simulink model "validate_magnetometer"  (R2014a)
settings: Solver=VariableStepDiscrete  StartTime=0.0  StopTime=t_sim  MaxStep=0.001  RelTol=1e-3
undefined symbols (not defined in the file): acc_data, diff, gravity_I, magnetometer_data, R_acc, R_magnetometer, ref_B_I
libraries: lib_gyro_fusion x7
settings Model: Creator=kirill  LastModifiedBy=kirill

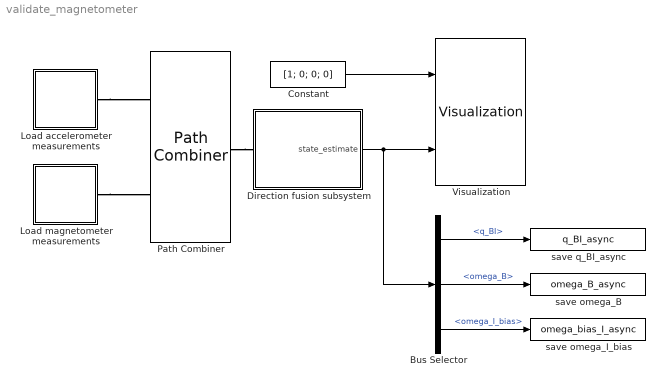
== system validate_magnetometer ==
  Bus Selector : BusSelector  OutputSignals=q_BI,omega_B,omega_I_bias
  Constant : Constant  Value=[1; 0; 0; 0]
  Direction fusion subsystem : Subsystem
  Load accelerometer measurements : Subsystem  mask{measurement_type=2, observed_data=acc_data, R_measurement=R_acc, ref_direction_I=gravity_I}
      mask prompts: measurement_type "Measuerment type (integer identifyer)"; observed_data "Observation data (see from workspace documentation)"; R_measurement "Measurement covariance matrix"; ref_direction_I "Reference direction"
  Load magnetometer measurements : Subsystem  mask{measurement_type=2, observed_data=magnetometer_data, R_measurement=R_magnetometer, ref_direction_I=ref_B_I}
      mask prompts: measurement_type "Measuerment type (integer identifyer)"; observed_data "Observation data (see from workspace documentation)"; R_measurement "Measurement covariance matrix"; ref_direction_I "Reference direction"
  Path Combiner : PathCombiner  NumberInputPorts=2
  Visualization : lib_gyro_fusion/Visualization
  save omega_B : ToWorkspace  VariableName=omega_B_async  SaveFormat=Timeseries  SampleTime=-1
  save omega_I_bias : ToWorkspace  VariableName=omega_bias_I_async  SaveFormat=Timeseries  SampleTime=-1
  save q_BI_async : ToWorkspace  VariableName=q_BI_async  SaveFormat=Timeseries  SampleTime=-1
  wires:
  Direction fusion subsystem/1(state_estimate) -> Visualization/2, Bus Selector/1
  Constant/1 -> Visualization/1
  Bus Selector/1 -> save q_BI_async/1  "<q_BI>"
  Bus Selector/3 -> save omega_I_bias/1  "<omega_I_bias>"
  Bus Selector/2 -> save omega_B/1  "<omega_B>"
  connections:
  Load accelerometer measurements/RConn1 -- Path Combiner/LConn1
  Path Combiner/RConn1 -- Direction fusion subsystem/LConn1
  Load magnetometer measurements/RConn1 -- Path Combiner/LConn2

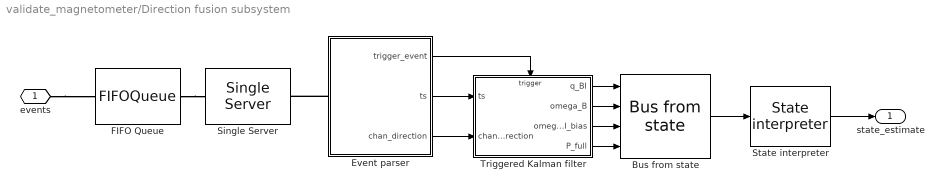
== system validate_magnetometer/Direction fusion subsystem ==
  Bus from state : lib_gyro_fusion/Bus from state
  Event parser : Subsystem
  FIFO Queue : FIFOQueue  Capacity=500
  Single Server : SingleServer  ServiceTime=0.001
  State interpreter : lib_gyro_fusion/State interpreter
  Triggered Kalman filter : Subsystem  TreatAsAtomicUnit=on
  events : PMIOPort  Port=1  Side=Left
  state_estimate : Outport
  wires:
  Event parser/3(chan_direction) -> Triggered Kalman filter/2(chan_direction)
  Event parser/1(trigger_event) -> Triggered Kalman filter/Trigger
  Event parser/2(ts) -> Triggered Kalman filter/1(ts)
  Bus from state/1 -> State interpreter/1
  State interpreter/1 -> state_estimate/1
  Triggered Kalman filter/1(q_BI) -> Bus from state/1
  Triggered Kalman filter/2(omega_B) -> Bus from state/2
  Triggered Kalman filter/3(omega_I_bias) -> Bus from state/3
  Triggered Kalman filter/4(P_full) -> Bus from state/4
  connections:
  events/RConn1 -- FIFO Queue/LConn1
  FIFO Queue/RConn1 -- Single Server/LConn1
  Event parser/LConn1 -- Single Server/RConn1

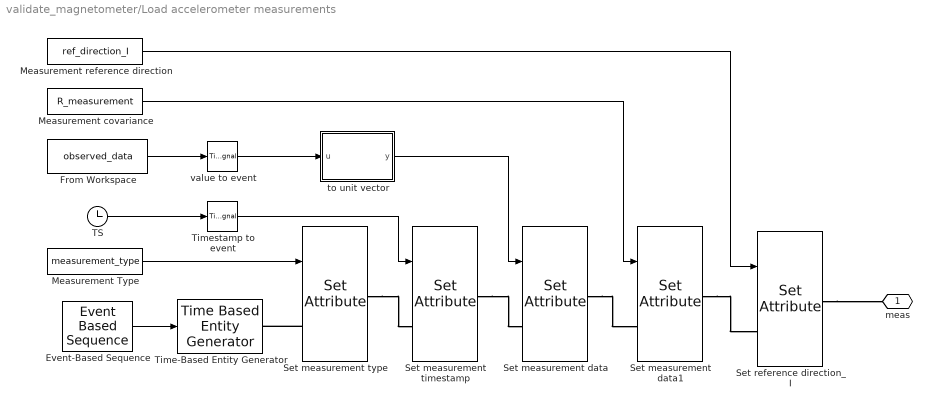
== system validate_magnetometer/Load accelerometer measurements ==
  Event-Based Sequence : EventBasedSequence  VectorOutputValues=diff(observed_data.time)  FormOutputOpt=Setting to infinity
  From Workspace : FromWorkspace  VariableName=observed_data  SampleTime=0
  Measurement Type : Constant  Value=measurement_type
  Measurement covariance : Constant  Value=R_measurement
  Measurement reference direction : Constant  Value=ref_direction_I
  Set measurement data : SetAttribute  AttributeName=value  AttributeFrom=Signal port  EvaluatedAttributeValue={ []}
  Set measurement data1 : SetAttribute  AttributeName=R  AttributeFrom=Signal port  EvaluatedAttributeValue={ []}
  Set measurement timestamp : SetAttribute  AttributeName=ts  AttributeFrom=Signal port  EvaluatedAttributeValue={ []}
  Set measurement type : SetAttribute  AttributeName=meas_type  AttributeFrom=Signal port  EvaluatedAttributeValue={ []}
  Set reference direction_I : SetAttribute  AttributeName=ref_direction_I  AttributeFrom=Signal port  EvaluatedAttributeValue={ []}
  TS : Clock
  Time-Based Entity Generator : TimeBasedEntityGenerator  GenerateEntitiesUpon=Intergeneration time from port t
  Timestamp to event : TimedToEventSignal
  to unit vector : MATLAB Function  TreatAsAtomicUnit=on
  value to event : TimedToEventSignal
  meas : PMIOPort  Port=1  Side=Right
  wires:
  TS/1 -> Timestamp to event/1
  From Workspace/1 -> value to event/1
  Event-Based Sequence/1 -> Time-Based Entity Generator/1
  Measurement Type/1 -> Set measurement type/1
  Timestamp to event/1 -> Set measurement timestamp/1
  value to event/1 -> to unit vector/1(u)
  Measurement covariance/1 -> Set measurement data1/1
  Measurement reference direction/1 -> Set reference direction_I/1
  to unit vector/1(y) -> Set measurement data/1
  connections:
  Set measurement type/LConn1 -- Time-Based Entity Generator/RConn1
  Set measurement type/RConn1 -- Set measurement timestamp/LConn1
  Set measurement timestamp/RConn1 -- Set measurement data/LConn1
  Set measurement data/RConn1 -- Set measurement data1/LConn1
  Set measurement data1/RConn1 -- Set reference direction_I/LConn1
  Set reference direction_I/RConn1 -- meas/RConn1

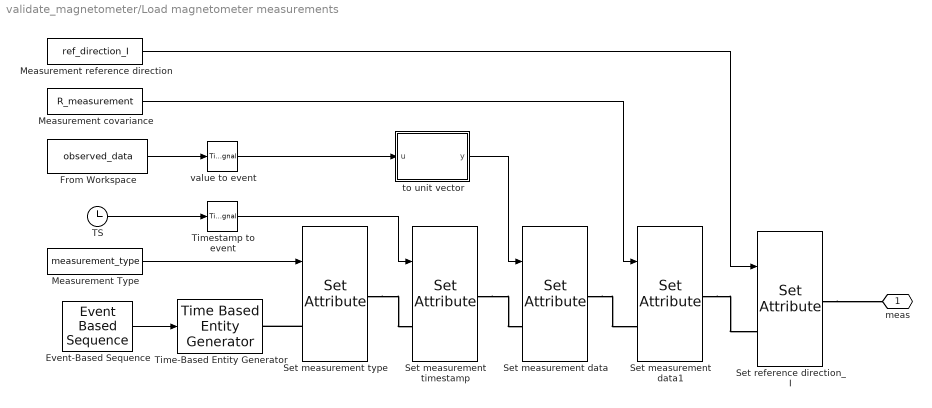
== system validate_magnetometer/Load magnetometer measurements ==
  Event-Based Sequence : EventBasedSequence  VectorOutputValues=diff(observed_data.time)  FormOutputOpt=Setting to infinity
  From Workspace : FromWorkspace  VariableName=observed_data  SampleTime=0
  Measurement Type : Constant  Value=measurement_type
  Measurement covariance : Constant  Value=R_measurement
  Measurement reference direction : Constant  Value=ref_direction_I
  Set measurement data : SetAttribute  AttributeName=value  AttributeFrom=Signal port  EvaluatedAttributeValue={ []}
  Set measurement data1 : SetAttribute  AttributeName=R  AttributeFrom=Signal port  EvaluatedAttributeValue={ []}
  Set measurement timestamp : SetAttribute  AttributeName=ts  AttributeFrom=Signal port  EvaluatedAttributeValue={ []}
  Set measurement type : SetAttribute  AttributeName=meas_type  AttributeFrom=Signal port  EvaluatedAttributeValue={ []}
  Set reference direction_I : SetAttribute  AttributeName=ref_direction_I  AttributeFrom=Signal port  EvaluatedAttributeValue={ []}
  TS : Clock
  Time-Based Entity Generator : TimeBasedEntityGenerator  GenerateEntitiesUpon=Intergeneration time from port t
  Timestamp to event : TimedToEventSignal
  to unit vector : MATLAB Function  TreatAsAtomicUnit=on
  value to event : TimedToEventSignal
  meas : PMIOPort  Port=1  Side=Right
  wires:
  TS/1 -> Timestamp to event/1
  From Workspace/1 -> value to event/1
  Event-Based Sequence/1 -> Time-Based Entity Generator/1
  Measurement Type/1 -> Set measurement type/1
  Timestamp to event/1 -> Set measurement timestamp/1
  value to event/1 -> to unit vector/1(u)
  Measurement covariance/1 -> Set measurement data1/1
  Measurement reference direction/1 -> Set reference direction_I/1
  to unit vector/1(y) -> Set measurement data/1
  connections:
  Set measurement type/LConn1 -- Time-Based Entity Generator/RConn1
  Set measurement type/RConn1 -- Set measurement timestamp/LConn1
  Set measurement timestamp/RConn1 -- Set measurement data/LConn1
  Set measurement data/RConn1 -- Set measurement data1/LConn1
  Set measurement data1/RConn1 -- Set reference direction_I/LConn1
  Set reference direction_I/RConn1 -- meas/RConn1

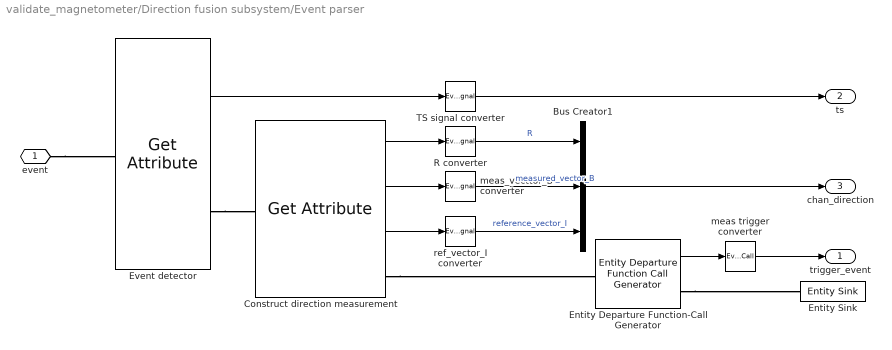
== system validate_magnetometer/Direction fusion subsystem/Event parser ==
  Bus Creator1 : BusCreator  Inputs=3
  Construct direction measurement : GetAttribute  AttributeName=R|value|ref_direction_I  AttributeMissing=Error|Error|Error  AttributeDefaultValue=1|1|1  AttributeTreatAsVector=1|1|1  AttributeSendTiming=After entity departure|After entity departure|After entity departure  EvaluatedDefaultAttributeValue={ [];[];[]}
      settings: OutputPortMap=o1,o2,o3
  Entity Departure Function-Call Generator : EntityDepartureFunctionCallGenerator
  Entity Sink : EntitySink
  Event detector : GetAttribute  AttributeName=ts  EvaluatedDefaultAttributeValue={ []}
      settings: OutputPortMap=o1
  R converter : EventToTimedSignal
  TS signal converter : EventToTimedSignal
  meas trigger converter : EventToTimedFunctionCall
  meas_vecttor_B converter : EventToTimedSignal
  ref_vector_I converter : EventToTimedSignal
  event : PMIOPort  Port=1  Side=Left
  trigger_event : Outport
  ts : Outport  Port=2
  chan_direction : Outport  Port=3
  wires:
  Construct direction measurement/1 -> R converter/1
  Bus Creator1/1 -> chan_direction/1
  Construct direction measurement/2 -> meas_vecttor_B converter/1
  ref_vector_I converter/1 -> Bus Creator1/3  "reference_vector_I"
  R converter/1 -> Bus Creator1/1  "R"
  meas_vecttor_B converter/1 -> Bus Creator1/2  "measured_vector_B"
  Construct direction measurement/3 -> ref_vector_I converter/1
  Entity Departure Function-Call Generator/1 -> meas trigger converter/1
  meas trigger converter/1 -> trigger_event/1
  TS signal converter/1 -> ts/1
  Event detector/1 -> TS signal converter/1
  connections:
  Entity Departure Function-Call Generator/RConn1 -- Entity Sink/LConn1
  Construct direction measurement/RConn1 -- Entity Departure Function-Call Generator/LConn1
  event/RConn1 -- Event detector/LConn1
  Event detector/RConn1 -- Construct direction measurement/LConn1

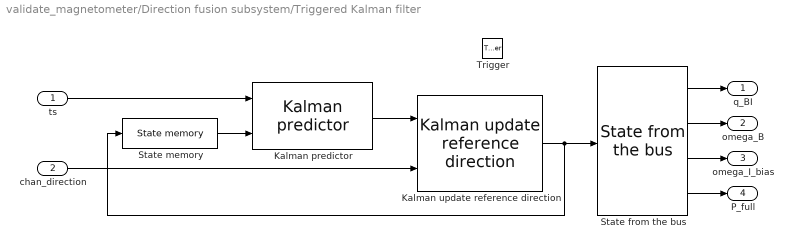
== system validate_magnetometer/Direction fusion subsystem/Triggered Kalman filter ==
  ts : Inport
  chan_direction : Inport  Port=2
  Trigger : TriggerPort  TriggerType=function-call
  Kalman predictor : lib_gyro_fusion/Kalman predictor  q_noise=q_noise  omega_B_noise=omega_B_noise  omega_I_bias_noise=omega_bias_I_noise
  Kalman update reference direction : lib_gyro_fusion/Kalman update reference direction
  State from the bus : lib_gyro_fusion/State from the bus
  State memory : lib_gyro_fusion/State memory  q_BI_init=[1; 0; 0; 0]  omega_B_init=[0; 0; 0]  omega_I_bias_init=[0; 0; 0]  P_full_init=eye(9)
  q_BI : Outport
  omega_B : Outport  Port=2
  omega_I_bias : Outport  Port=3
  P_full : Outport  Port=4
  wires:
  ts/1 -> Kalman predictor/1
  chan_direction/1 -> Kalman update reference direction/2
  State memory/1 -> Kalman predictor/2
  Kalman update reference direction/1 -> State memory/1, State from the bus/1
  Kalman predictor/1 -> Kalman update reference direction/1
  State from the bus/1 -> q_BI/1
  State from the bus/2 -> omega_B/1
  State from the bus/3 -> omega_I_bias/1
  State from the bus/4 -> P_full/1

== matlab function validate_magnetometer/Load magnetometer measurements/to unit vector ==
  data: u input; y output
function y = to_unit(u)
%#codegen

y = u / norm(u);

== matlab function validate_magnetometer/Load accelerometer measurements/to unit vector ==
  data: u input; y output
function y = to_unit(u)
%#codegen

y = u / norm(u);
